simulink model "step_14"  (R2014b)
settings: Solver=ode45  StartTime=0.0  StopTime=10.0  RelTol=1e-3
values from neighbouring files (symbols this model uses):
  B = sys.b    [MinSeg_Parameters.m]    (also in MinSeg_Parameters_v2.m = [0; Brow2; 0; Brow3]; MinSeg_Parameters_v3.m = [0; Brow2; 0; Brow3])
  C = sys.c    [MinSeg_Parameters.m]    (also in MinSeg_Parameters_v2.m = eye(N); MinSeg_Parameters_v3.m = eye(N))
  D = sys.d    [MinSeg_Parameters.m]    (also in MinSeg_Parameters_v2.m = zeros(N, 1); MinSeg_Parameters_v3.m = zeros(N, 1))
undefined symbols (not defined in the file or in its folder): Acl, xini
settings Model: Creator=mo114c  LastModifiedBy=mo114c
settings DebuggingCC: UnderspecifiedInitializationDetection=Classic  MergeDetectMultiDrivingBlocksExec=none  SolverPrmCheckMsg=none  StateNameClashWarn=warning

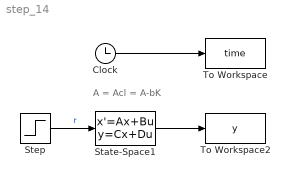
== system step_14 ==
  note: A = Acl = A-bK
  Clock : Clock
  State-Space1 : StateSpace  A=Acl  B=B  C=C  D=D  X0=xini
  Step : Step  SampleTime=0
  To Workspace : ToWorkspace  VariableName=time  SampleTime=-1
  To Workspace2 : ToWorkspace  VariableName=y  SampleTime=-1
  wires:
  Clock/1 -> To Workspace/1
  State-Space1/1 -> To Workspace2/1
  Step/1 -> State-Space1/1  "r"
